simulink model "DirectConversionReciever"  (R2015b)
settings: Solver=VariableStepAuto  StartTime=0.0  StopTime=10.0  RelTol=1e-3
libraries: rfmathmodels1 x4, simulink x2, simrfV2elements x2, commrflib2 x1, dspxfrm3 x1, dspvision x1, commanabbnd3 x1
settings Model: Creator=dominikguz  LastModifiedBy=dominikguz

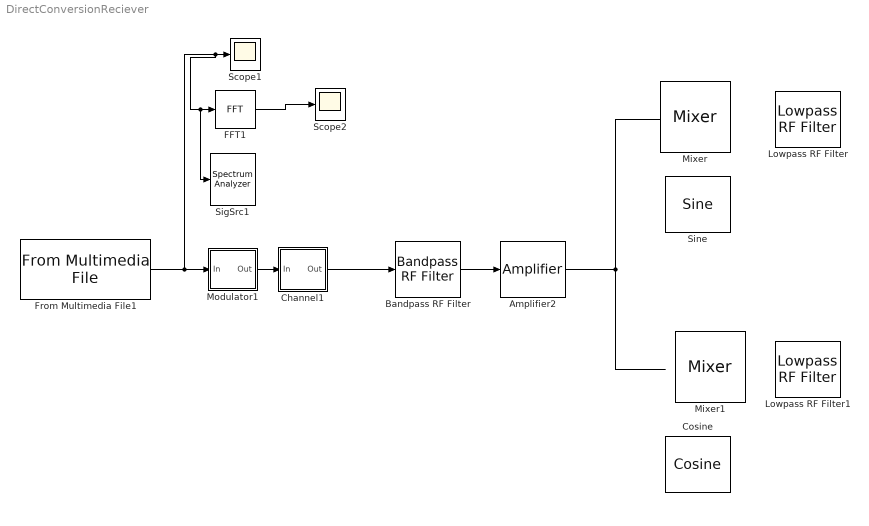
== system DirectConversionReciever ==
  Amplifier2 : rfmathmodels1/Amplifier  model_select=Linear  linGaindB=0  GindB=0  iip3=30  am2pm=10  PwrAMPMStart=10  PwrAMPMEnd=inf  amam=[2.1587 1.1517]  ampm=[4.0033 9.1040]  x=[8.1081 1.5413 6.5202 -0.0718]  y=[4.6645 2.0965 10.88 -0.003]  p=0.5  GoutdB=0  vsat=1  method_select=Noise factor  ntemp=290  nfigure=3.01  nfactor=2  seed=67987
  Bandpass RF Filter : rfmathmodels1/Bandpass RF Filter  method=Butterworth  filttype=Bandpass  N=3  flo=1.9998e9  fhi=2.0002e9  Rp=1  Rs=10  MaxLength=32  Fc=2e9  Ts=1e-6
  Channel1 : Subsystem
  Cosine : simulink/Lookup Tables/Cosine  Formula=cos(2*pi*u)  NumDataPoints=(2^5)+1  OutputWordLength=16  InternalRulePriority=Speed
  FFT1 : dspxfrm3/FFT  FFTImplementation=Auto  CompMethod=Table lookup  TableOpt=NEW  TableOptActive=Speed  BitRevOrder=off  Normalize=off  InheritFFTLength=on  FFTLength=64  WrapInput=on  roundingMode=Floor  overflowMode=off  firstCoeffDataTypeStr=Inherit: Same word length as input  firstCoeffLastDataTypeStr=Inherit: Same word length as input  outputMin=[]  outputMax=[]
  From Multimedia File1 : dspvision/From Multimedia File  inputFilename=guitartune.wav  loop=on  numPlays=1  outputStreams=Audio only  videoDataType=single  audioDataType=double  inheritSampleTime=on  userDefinedSampleTime=1/4410  noAudioOutput=off  isIntensityVideo=off  fourcc=RGB  colorVideoFormat=Separate color signals  outputEOF=off  dataOrg=Column-major  audioFrameSize=4410  computeAudioFrameSize=off  outSamplingMode=Sample based
  Lowpass RF Filter : rfmathmodels1/Lowpass RF Filter  method=Butterworth  filttype=Lowpass  N=3  flo=1.9998e9  fhi=2.0002e9  Rp=1  Rs=10  MaxLength=32  Fc=2e9  Ts=1e-6
  Lowpass RF Filter1 : rfmathmodels1/Lowpass RF Filter  method=Butterworth  filttype=Lowpass  N=3  flo=1.9998e9  fhi=2.0002e9  Rp=1  Rs=10  MaxLength=32  Fc=2e9  Ts=1e-6
  Mixer : simrfV2elements/Mixer  classname=mixer  Source_linear_gain=Available power gain  linear_gain=0 dB  Zin=50  Zout=50  ZLO=inf  Source_Poly=Even and odd order  Poly_Coeffs=[0 1]  IPType=Output  IP2=Inf dBm  IP3=Inf dBm  P1dB=Inf dBm  Psat=Inf dBm  Gcomp=Inf dBm  NF=0  InternalGrounding=on
  Mixer1 : simrfV2elements/Mixer  classname=mixer  Source_linear_gain=Available power gain  linear_gain=0 dB  Zin=50  Zout=50  ZLO=inf  Source_Poly=Even and odd order  Poly_Coeffs=[0 1]  IPType=Output  IP2=Inf dBm  IP3=Inf dBm  P1dB=Inf dBm  Psat=Inf dBm  Gcomp=Inf dBm  NF=0  InternalGrounding=on
  Modulator1 : Subsystem
  Scope1 : Scope
  Scope2 : Scope
  SigSrc1 : SpectrumAnalyzer
  Sine : simulink/Lookup Tables/Sine  Formula=sin(2*pi*u)  NumDataPoints=(2^5)+1  OutputWordLength=16  InternalRulePriority=Speed
  wires:
  Bandpass RF Filter/1 -> Amplifier2/1
  Modulator1/1(Out) -> Channel1/1(In)
  Channel1/1(Out) -> Bandpass RF Filter/1
  From Multimedia File1/1 -> SigSrc1/1, FFT1/1, Scope1/1, Modulator1/1(In)
  FFT1/1 -> Scope2/1
  Amplifier2/1 -> ?
  ? -> Lowpass RF Filter1/1
  ? -> Lowpass RF Filter/1

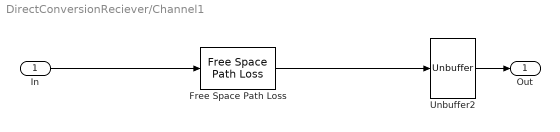
== system DirectConversionReciever/Channel1 ==
  In : Inport
  Free Space Path Loss : commrflib2/Free Space Path Loss  mode=Decibels  dB=120  d=0.100  fc=1920
  Unbuffer2 : Unbuffer  SampleBasedProcessing=Same as frame based
  Out : Outport
  wires:
  Free Space Path Loss/1 -> Unbuffer2/1
  Unbuffer2/1 -> Out/1
  In/1 -> Free Space Path Loss/1

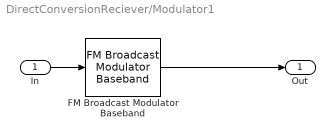
== system DirectConversionReciever/Modulator1 ==
  In : Inport
  FM Broadcast Modulator Baseband : commanabbnd3/FM Broadcast Modulator Baseband  SampleRate=152e3  FrequencyDeviation=75e3  FilterTimeConstant=75e-6  AudioSampleRate=44100  Stereo=off  SimulateUsing=Code generation
  Out : Outport
  wires:
  In/1 -> FM Broadcast Modulator Baseband/1
  FM Broadcast Modulator Baseband/1 -> Out/1
